simulink model "first"  (R2021b)
settings: Solver=VariableStepAuto  StartTime=0.0  StopTime=10.0  RelTol=1e-3
undefined symbols (not defined in the file): Ion, Lithium
libraries: spsDiodeLib x8, spsMosfetLib x8, spsSeriesRLCBranchLib x8, spsACVoltageSourceLib x1, spsBatteryLib x1, spsMultiWindingTransformerLib x1, spsSawtoothGeneratorLib x1, spsVoltageMeasurementLib x1, spspowerguiLib x1
settings Model: Creator=eee  LastModifiedBy=eee

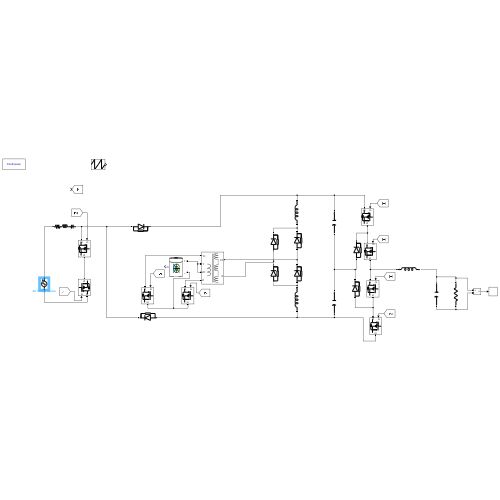
[thumbnail: Simulink's stored preview of the top-level diagram]
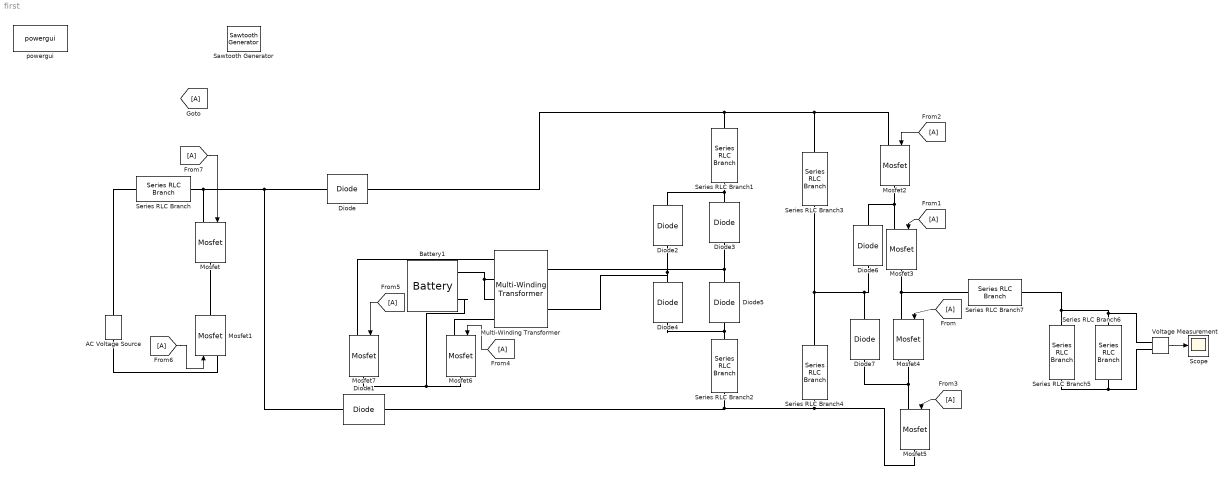
== system first ==
  AC Voltage Source : spsACVoltageSourceLib/AC Voltage Source  Amplitude=100  Phase=0  Frequency=60  SampleTime=0  Measurements=None  BusType=swing  Pref=10e3  Qref=0  Qmin=-inf  Qmax=+inf
  Battery1 : spsBatteryLib/Battery  BatType=Lithium-Ion  ShowTempParam=off  ThermalPreset=no  ShowAgeParam=off  NomV=7.2  NomQ=5.4  SOC=100  Batt_Tr=30  PresetModel=on  MaxQ=5.4  MinV=5.4  FullV=8.3807  Dis_rate=2.3478  R=0.013333  Normal_OP=4.8835  expZone="[7.7788      0.2653]"  current=[6.5 13 32.5]  Units=Time  Tci=20  NomT=20  T2=-30  MaxQ2=4.8  FullV2=7.1  Normal_OP2=5.655  expZone2="[6.58           1]"  Rca=0.6  ti=2000  Dp=0  Neq0=0  Tsim=1e6  Ta1=25  Qeol=5.4*0.9  Reol=0.013333*1.2  Char_age=[2.3478, 3]  Dis_age=[2.3478, 10]  N1=1500  N2=10500  N3=1000  N4=1400  Ta2=45  N5=950
  Diode{,1..7} (8 alike) : spsDiodeLib/Diode  Ron=0.001  Lon=0  Vf=0.8  IC=0  UseSnubber=0  Rs=500  Cs=250e-9  Measurements=off
  Mosfet{,1..7} (8 alike) : spsMosfetLib/Mosfet  Ron=0.1  Lon=0  Rd=0.01  Vfd=0  IC=0  Rs=1e5  Cs=inf  Measurements=off
  Multi-Winding Transformer : spsMultiWindingTransformerLib/Multi-Winding Transformer  LeftWindings=2  RightWindings=1  TappedWindings=no taps  NumberOfTaps=2  SetSaturation=off  Hysteresis=off  DataFile='hysteresis.mat'  Measurements=None  UNITS=pu  NominalPower=[75e3 60]  NominalVoltages="[ 14400  120  120 120 ]"  WindingResistances="[ 0.005  0.005  0.005  0.005]"  WindingInductances="[ 0.02  0.02  0.02  0.02 ]"  Rm=50  Lm=50  Saturation=[ 0,0 ; 0.0024,1.2 ; 1.0,1.52 ]  BreakLoop=off  DiscreteSolver=Trapezoidal iterative  DataType=off  InitialFlux=0  TransfoNumber=1
      settings: SourceProductBaseCode=PS
  Sawtooth Generator : spsSawtoothGeneratorLib/Sawtooth Generator  Freq=1e3  Phase=180  Ts=0
  Scope : Scope
  Series RLC Branch : spsSeriesRLCBranchLib/Series RLC Branch  LConnTagsString=__new0  RConnTagsString=__new0  BranchType=RLC  Resistance=1  Inductance=1e-3  SetiL0=off  InitialCurrent=0  Capacitance=1e-6  Setx0=off  InitialVoltage=0  Measurements=None
  Series RLC Branch1 : spsSeriesRLCBranchLib/Series RLC Branch  LConnTagsString=__new0  RConnTagsString=__new0  BranchType=L  Resistance=1  Inductance=1e-3  SetiL0=off  InitialCurrent=0  Capacitance=1e-6  Setx0=off  InitialVoltage=0  Measurements=None
  Series RLC Branch2 : spsSeriesRLCBranchLib/Series RLC Branch  LConnTagsString=__new0  RConnTagsString=__new0  BranchType=L  Resistance=1  Inductance=1e-3  SetiL0=off  InitialCurrent=0  Capacitance=1e-6  Setx0=off  InitialVoltage=0  Measurements=None
  Series RLC Branch3 : spsSeriesRLCBranchLib/Series RLC Branch  LConnTagsString=__new0  RConnTagsString=__new0  BranchType=C  Resistance=1  Inductance=1e-3  SetiL0=off  InitialCurrent=0  Capacitance=1e-6  Setx0=off  InitialVoltage=0  Measurements=None
  Series RLC Branch4 : spsSeriesRLCBranchLib/Series RLC Branch  LConnTagsString=__new0  RConnTagsString=__new0  BranchType=C  Resistance=1  Inductance=1e-3  SetiL0=off  InitialCurrent=0  Capacitance=1e-6  Setx0=off  InitialVoltage=0  Measurements=None
  Series RLC Branch5 : spsSeriesRLCBranchLib/Series RLC Branch  LConnTagsString=__new0  RConnTagsString=__new0  BranchType=C  Resistance=1  Inductance=1e-3  SetiL0=off  InitialCurrent=0  Capacitance=1e-6  Setx0=off  InitialVoltage=0  Measurements=None
  Series RLC Branch6 : spsSeriesRLCBranchLib/Series RLC Branch  LConnTagsString=__new0  RConnTagsString=__new0  BranchType=R  Resistance=1  Inductance=1e-3  SetiL0=off  InitialCurrent=0  Capacitance=1e-6  Setx0=off  InitialVoltage=0  Measurements=None
  Series RLC Branch7 : spsSeriesRLCBranchLib/Series RLC Branch  LConnTagsString=__new0  RConnTagsString=__new0  BranchType=L  Resistance=1  Inductance=1e-3  SetiL0=off  InitialCurrent=0  Capacitance=1e-6  Setx0=off  InitialVoltage=0  Measurements=None
  Voltage Measurement : spsVoltageMeasurementLib/Voltage Measurement  PhasorSimulation=off  OutputType=Complex  PSBequivalent=0
  powergui : spspowerguiLib/powergui  Priority=1  SimulationMode=Continuous  SampleTime=50e-6  frequency=60  Iterations=50  frequencyindice=60  Pbase=100e6  ErrMax=1e-4  UnitsV=kV  UnitsW=MW  buscounter=0  FunctionMessages=off  echomessages=off  EnableUseOfTLC=off  CurrentSourceSwitches=off  DisableSnubberDevices=off  DisableRonSwitches=off  DisableVfSwitches=off  DisplayEquations=off  AutomaticDiscreteSolvers=off  SolverType=Tustin/Backward Euler (TBE)  Interpol=off  ExternalGateDelay=off  methode=off  Ts=100  x0status=blocks  SPID=on  SwTol=0  HookPort=off  NonlinearTolerance=1e-4  nMaxIteration=100  ContinueOnMaxIteration=off  RestoreLinks=warning  ResistiveCurrentMeasurement=off  Frange=[0:2:500]  Ylog=off  Xlog=on  ShowGrid=off  save=off  variable=ZData  structure=0  ZoomFFT=off  StartTime=0.0  cycles=1  DisplayStyle=1  fundamental=60  FreqAxis=off  MaxFrequency=1000  frequencyindicesteady=1  RmsSteady=1  display=off
  wires:
  Voltage Measurement/1 -> Scope/1
  [A] -> Mosfet4/1
  [A] -> Mosfet/1
  [A] -> Mosfet1/1
  [A] -> Mosfet7/1
  [A] -> Mosfet6/1
  [A] -> Mosfet3/1
  [A] -> Mosfet2/1
  [A] -> Mosfet5/1
  connections:
  AC Voltage Source/RConn1 -- Series RLC Branch/LConn1
  Mosfet/RConn1 -- Mosfet1/RConn1
  Series RLC Branch/RConn1 -- Diode1/RConn1 -- Diode/LConn1 -- Mosfet/LConn1
  Mosfet1/LConn1 -- AC Voltage Source/LConn1
  Series RLC Branch1/RConn1 -- Diode2/RConn1 -- Diode3/RConn1
  Series RLC Branch2/LConn1 -- Diode4/LConn1 -- Diode5/LConn1
  Diode3/LConn1 -- Multi-Winding Transformer/RConn1 -- Diode5/RConn1
  Diode2/LConn1 -- Multi-Winding Transformer/RConn2 -- Diode4/RConn1
  Diode1/LConn1 -- Mosfet5/RConn1 -- Series RLC Branch4/RConn1 -- Series RLC Branch2/RConn1
  Diode/RConn1 -- Mosfet2/LConn1 -- Series RLC Branch3/LConn1 -- Series RLC Branch1/LConn1
  Mosfet2/RConn1 -- Diode6/RConn1 -- Mosfet3/LConn1
  Mosfet3/RConn1 -- Mosfet4/LConn1 -- Series RLC Branch7/LConn1
  Mosfet4/RConn1 -- Diode7/LConn1 -- Mosfet5/LConn1
  Diode7/RConn1 -- Series RLC Branch3/RConn1 -- Series RLC Branch4/LConn1 -- Diode6/LConn1
  Series RLC Branch5/LConn1 -- Voltage Measurement/LConn1 -- Series RLC Branch6/LConn1 -- Series RLC Branch7/RConn1
  Series RLC Branch6/RConn1 -- Voltage Measurement/LConn2 -- Series RLC Branch5/RConn1
  Multi-Winding Transformer/LConn2 -- Multi-Winding Transformer/LConn3 -- Battery1/LConn1
  Mosfet7/RConn1 -- Battery1/LConn2 -- Mosfet6/RConn1
  Mosfet6/LConn1 -- Multi-Winding Transformer/LConn4
  Mosfet7/LConn1 -- Multi-Winding Transformer/LConn1
